simulink subsystem "accCM2Sensor"  (R2021a)
settings: Solver=VariableStepAuto  StartTime=0.0  StopTime=10.0  RelTol=1e-3
undefined symbols (not defined in the file): config
libraries: attitude_library x5, vrlib x3
settings Model: Creator=Laura  LastModifiedBy=Laura

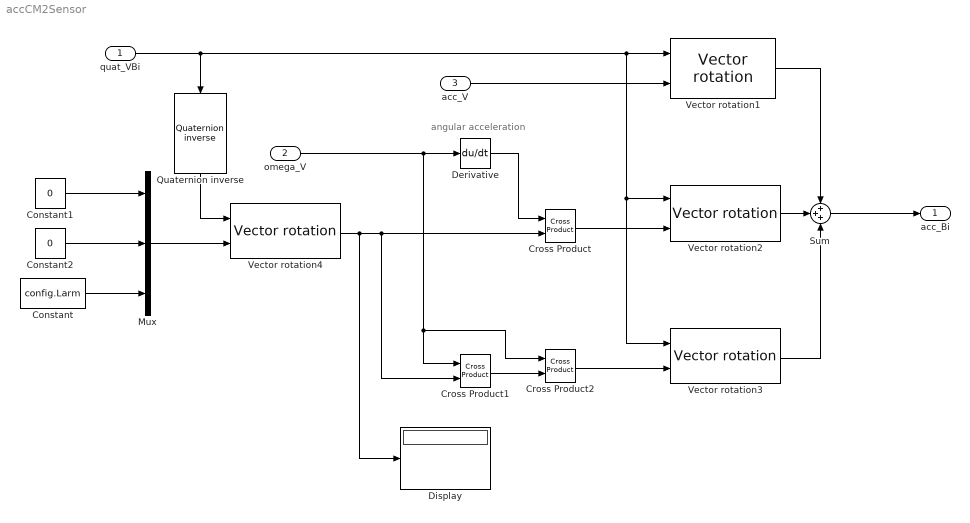
== system accCM2Sensor ==
  note: angular acceleration
  quat_VBi : Inport
  omega_V : Inport  Port=2
  acc_V : Inport  Port=3
  Constant : Constant  Value=config.Larm
  Constant1 : Constant  Value=0
  Constant2 : Constant  Value=0
  Cross Product : vrlib/Utilities/Cross Product
  Cross Product1 : vrlib/Utilities/Cross Product
  Cross Product2 : vrlib/Utilities/Cross Product
  Derivative : Derivative
  Display : Display
  Mux : Mux  Inputs=3
  Quaternion inverse : attitude_library/Quaternion inverse  SystemSampleTime=-1  VariantActivationTime=update diagram  Latency=0  AutoFrameSizeCalculation=off
      settings: SourceProductName=Attitude library
  Sum : Sum  Inputs=+++
  Vector rotation{1..4} (4 alike) : attitude_library/Vector rotation  SystemSampleTime=-1  VariantActivationTime=update diagram  Latency=0  AutoFrameSizeCalculation=off
      settings: SourceProductName=Attitude library
  acc_Bi : Outport
  wires:
  Quaternion inverse/1 -> Vector rotation4/1
  Vector rotation2/1 -> Sum/2
  Cross Product/1 -> Vector rotation2/2
  Derivative/1 -> Cross Product/1
  Mux/1 -> Vector rotation4/2
  Vector rotation4/1 -> Cross Product/2, Cross Product1/2, Display/1
  Vector rotation1/1 -> Sum/1
  Constant2/1 -> Mux/2
  acc_V/1 -> Vector rotation1/2
  omega_V/1 -> Derivative/1, Cross Product2/1, Cross Product1/1
  Constant/1 -> Mux/3
  Constant1/1 -> Mux/1
  quat_VBi/1 -> Quaternion inverse/1, Vector rotation1/1, Vector rotation3/1, Vector rotation2/1
  Cross Product1/1 -> Cross Product2/2
  Sum/1 -> acc_Bi/1
  Vector rotation3/1 -> Sum/3
  Cross Product2/1 -> Vector rotation3/2
